simulink model "VABSim_non_lin"  (R2019b)
settings: Solver=VariableStepAuto  StartTime=0.0  StopTime=10.0  RelTol=1e-3
values from neighbouring files (symbols this model uses):
  coeffs_den = double(coeffs(den,'all'))    [fdt_vab_lineare.m]
  coeffs_num = double(coeffs(num,'all'))    [fdt_vab_lineare.m]
undefined symbols (not defined in the file or in its folder): control_on, k_p, sigbuilder_block, theta_secondo
settings Model: Creator=AndreaCalegari  LastModifiedBy=AndreaCalegari

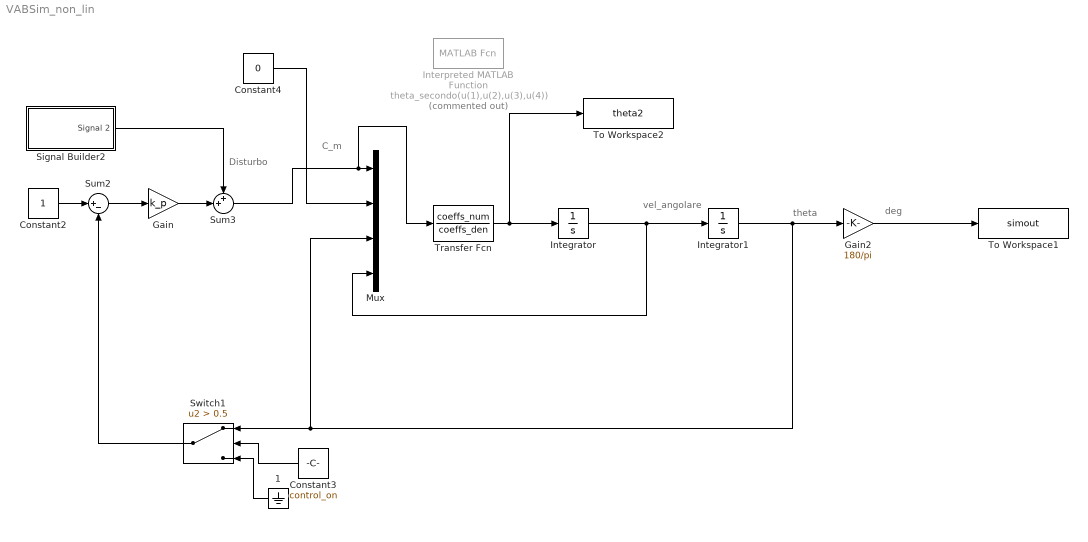
== system VABSim_non_lin ==
  note: Disturbo
  note: theta
  note: C_m
  note: deg
  note: vel_angolare
  " 1" : Ground
  Constant2 : Constant
  Constant3 : Constant  Value=control_on
  Constant4 : Constant  Value=0
  Gain : Gain  Gain=k_p
  Gain2 : Gain  Gain=180/pi  OutMin=[-180]  OutMax=[+180]
  Integrator : Integrator
  Integrator1 : Integrator
  Interpreted MATLAB Function : MATLABFcn  Commented=on  MATLABFcn=theta_secondo(u(1),u(2),u(3),u(4))  OutputDimensions=1
  Mux : Mux
  Signal Builder2 : Subsystem  Tag=STV Subsys  LoadFcn=sigbuilder_block('load');  StartFcn=sigbuilder_block('start');  StopFcn=sigbuilder_block('stop');  ClipboardFcn=sigbuilder_block('clipboard');  mask(Sigbuilder block){tuvar=[0:10]}
      mask help: Simulink:masks:SigbuilderBlock_MD
      mask init:
      | if ~strcmp(get_param(bdroot(gcbh),'SimulationStatus'),'stopped') tuvar = sigbuilder_block('maskInit'); end
      settings: CopyFcn=sigbuilder_block('copy');  DeleteFcn=sigbuilder_block('delete');  ModelCloseFcn=sigbuilder_block('modelClose');  PreSaveFcn=sigbuilder_block('preSave');  PauseFcn=sigbuilder_block('pause');  ContinueFcn=sigbuilder_block('continue');  NameChangeFcn=sigbuilder_block('namechange');  OpenFcn=sigbuilder_block('open',[6 25.5 1012.5 451.5 ]);  CloseFcn=sigbuilder_block('close');
      mask Display: plot(0, 0, 100, 100,[2, 2, 32, 32, 2], [68, 8, 8, 68, 68],[32, 2], [38, 38], [32, 19, 2],[53, 60, 44], [32, 17, 17, 2],[16, 16, 31, 31]);txt = getActiveGroup(gcbh);text(2, 100, txt,'verticalAlignment', 'top');
  Sum2 : Sum  Inputs=|+-
  Sum3 : Sum  Inputs=++|
  Switch1 : Switch  Criteria=u2 > Threshold  Threshold=0.5
  To Workspace1 : ToWorkspace  VariableName=simout  SaveFormat=Timeseries  SampleTime=-1
  To Workspace2 : ToWorkspace  VariableName=theta2  SaveFormat=Timeseries  SampleTime=-1
  Transfer Fcn : TransferFcn  Numerator=coeffs_num  Denominator=coeffs_den
  wires:
  Sum2/1 -> Gain/1
  Constant4/1 -> Mux/2
  " 1"/1 -> Switch1/3
  Sum3/1 -> Transfer Fcn/1, Mux/1
  Constant2/1 -> Sum2/1
  Integrator/1 -> Mux/4, Integrator1/1
  Gain2/1 -> To Workspace1/1
  Gain/1 -> Sum3/2
  Integrator1/1 -> Gain2/1, Mux/3, Switch1/1
  Signal Builder2/1(Signal 2) -> Sum3/1
  Switch1/1 -> Sum2/2
  Constant3/1 -> Switch1/2
  Transfer Fcn/1 -> To Workspace2/1, Integrator/1

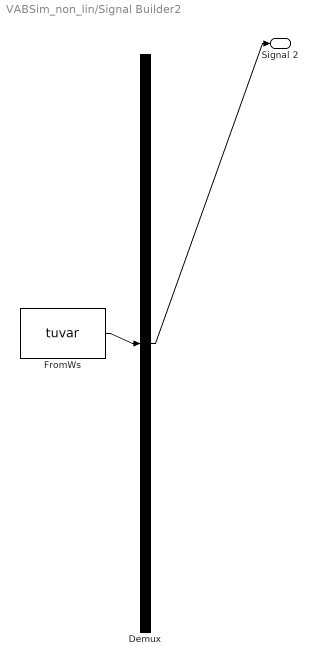
== system VABSim_non_lin/Signal Builder2 ==
  Demux : Demux  Tag=STV Demux  Outputs=1
  FromWs : FromWorkspace  Tag=STV FromWs  VariableName=tuvar  SampleTime=0
      SigBuilderData=|
      | common.afterFinalStr = 'Extrapolate'
      | common.sampleTime = 0
      | dataSet.timeRange = [0 20]
      | dataSet.name = 'Group 1'
      | sbobj.Groups.Name = 'Group 1'
      | sbobj.Groups.Signals.Name = 'Signal 2'
      | sbobj.Groups.Signals.XData = [0 1 1 1.86 1.86 20]
      | sbobj.Groups.Signals.YData = [0 0 4.9 4.9 0 0]
      | sbobj.Groups.TimeRange = [0 20]
  Signal 2 : Outport  Tag=STV Outport
  wires:
  FromWs/1 -> Demux/1
  Demux/1 -> Signal 2/1
